simulink model "simrewinder_scaled"  (R2023a)
settings: Solver=VariableStepAuto  StartTime=0.0  StopTime=200  RelTol=1e-3
values from neighbouring files (symbols this model uses):
  a = 25    [outperpi.m]    (also in rewinder_discrete.m)
  b = alpha*(a+Kt*Kv)    [outperpi.m]
  Keg = egv/egz    (= 3149.60629921)    [outperpi.m]
  Kl = 8/0.1    (= 80)    [outperpi.m]
  Kp = Kpmax*10^(log10(wc/wmax))    [outperpi.m]
  Kv = 20    [outperpi.m]
  Td = 0    [outperpi.m]
  umax = 5    [outperpi.m]
settings Model: Creator=mike_  LastModifiedBy=mike_
settings DataIOCC: ReturnWorkspaceOutputs=off
settings DebuggingCC: UnconnectedInputMsg=warning  UnconnectedOutputMsg=warning  UnconnectedLineMsg=warning
settings ModelReferenceCC: EnableRefExpFcnMdlSchedulingChecks=on
settings RTWCC: DLArmComputeVersion=19.05

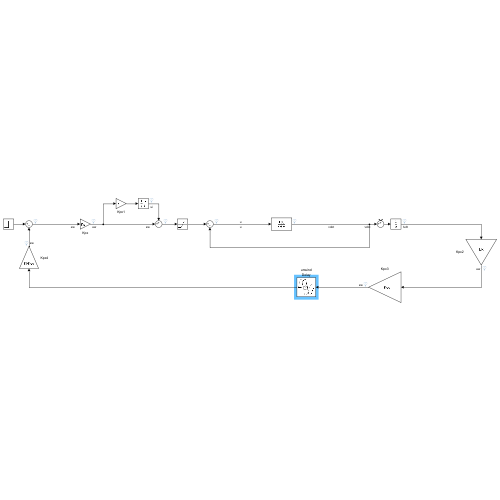
[thumbnail: Simulink's stored preview of the top-level diagram]
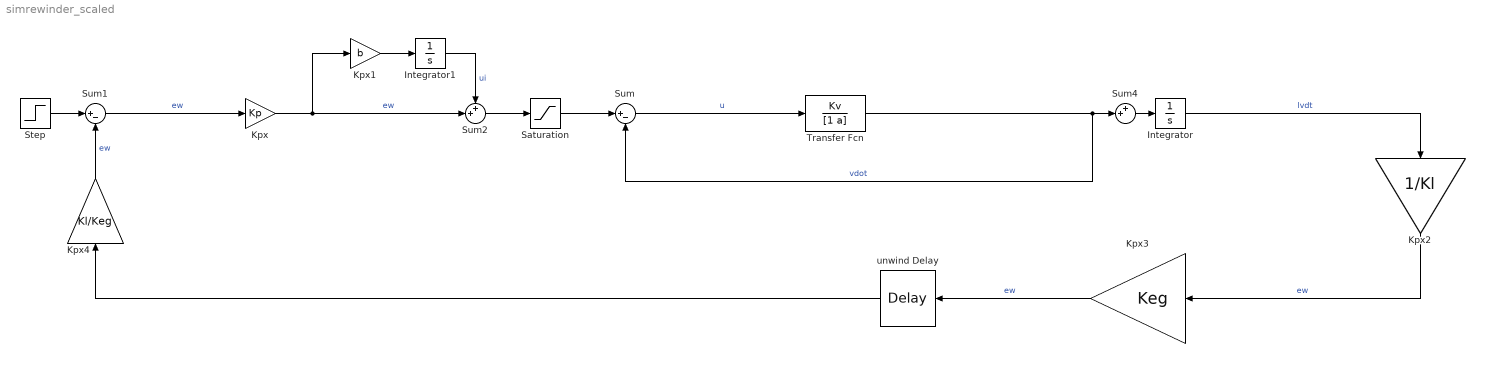
== system simrewinder_scaled ==
  Integrator : Integrator
  Integrator1 : Integrator  LimitOutput=on  UpperSaturationLimit=umax  LowerSaturationLimit=-umax
  Kpx : Gain  Gain=Kp
  Kpx1 : Gain  Gain=b
  Kpx2 : Gain  Gain=1/Kl
  Kpx3 : Gain  Gain=Keg
  Kpx4 : Gain  Gain=Kl/Keg
  Saturation : Saturate  UpperLimit=umax  LowerLimit=-umax
  Step : Step  Time=2  SampleTime=0
  Sum : Sum  Inputs=|+-
  Sum1 : Sum  Inputs=|+-
  Sum2 : Sum  Inputs=++|
  Sum4 : Sum  Inputs=++|
  Transfer Fcn : TransferFcn  Numerator=Kv  Denominator=[1 a]
  unwind Delay : TransportDelay  DelayTime=Td
  wires:
  Transfer Fcn/1 -> Sum4/2, Sum/2  "vdot"
  Step/1 -> Sum1/1
  unwind Delay/1 -> Kpx4/1
  Integrator/1 -> Kpx2/1  "lvdt"
  Sum/1 -> Transfer Fcn/1  "u"
  Sum4/1 -> Integrator/1
  Sum2/1 -> Saturation/1
  Kpx1/1 -> Integrator1/1
  Integrator1/1 -> Sum2/1  "ui"
  Kpx/1 -> Sum2/2, Kpx1/1  "ew"
  Saturation/1 -> Sum/1
  Kpx2/1 -> Kpx3/1  "ew"
  Sum1/1 -> Kpx/1  "ew"
  Kpx3/1 -> unwind Delay/1  "ew"
  Kpx4/1 -> Sum1/2  "ew"
